simulink model "TrajectoryFollowVehicleWith14DoF"  (R2024a)
settings: Solver=VariableStepAuto  StartTime=0  StopTime=14  FixedStep=timeStep  RelTol=1e-3
PreLoadFcn:
  | useDynamicsStanley = false; %Simulink model to move according to the scenario trajectory.
  | vehicleVariant = "3DOF";
PostLoadFcn:
  | load(fullfile(matlabroot,'toolbox','driving','drivingdata','rrScenarioSimTypes.mat'));
  | helperSLTrajectoryFollowerWithRRScenarioSetup();
  | heightMap = "flat";
  | if isfile("pathFollowingUtil/gridMap_groundHeight_RT.mat")
  |     load("gridMap_groundHeight_RT.mat");
  | end
  | % if exist("z_2DTable", "var") && exist("xBreakPts", "var") && exist("yBreakPts", "var")
  | %     hegihtMap = "2DMap";
  | % end
  | % if isfile("CRG/crgRoad.crg")
  | %     crgData = crg_read('CRG/crgRoad.crg');
  | % end
InitFcn:
  | if ~exist("useLongitudinalEV", "var")
  |     useLongitudinalEV = false;
  | end
StartFcn:
  | % set_param(bdroot, 'Profile', 'on');
StopFcn:
  | % set_param(bdroot, 'Profile', 'off');
  | % slprofreport(bdroot, 'report14DoF.html');
undefined symbols (not defined in the file or in its folder): ActorRuntime, Camera, control_timeStep, Defined, DiscIntNeverNeededParam, dz, Ego, egoInitialPose, egoInitialPoseCG, egoInitialPoseRear, InitVehicle, kmph2mps, Lane, lr, m, magnitude, max_dc, n, numReferencePose, pitch, roll, RRtimeStep, SceneData, SRE, steerGear, tau, tau2, timeStep, User, VehicleData, WheelPoses, X, xBreakPts, Y, yaw, yBreakPts, Z, z_2DTable
libraries: sm_lib x108, nesl_utility x62, sm_vehicle_utilities_lib x30, simulink_extras x12, roadrunnerscenario x6, simulink x4, drivingvehiclecontroller x4, autolibshared x2, mpcadaslib x2, autolibutils x1, METI_Lib_vehicle_model x1
(part 1 of 6)
settings Model: Creator=The MathWorks, Inc.  LastModifiedBy=nobuakif
settings DataIOCC: SaveOutput=off  DSMLogging=off  InspectSignalLogs=on  SaveTime=off  ReturnWorkspaceOutputs=off
settings OptimizationCC: DefaultParameterBehavior=Inlined  ReuseModelBlockBuffer=off
settings DebuggingCC: ParameterTunabilityLossMsg=error  UnconnectedInputMsg=warning  UnconnectedOutputMsg=warning  UnconnectedLineMsg=warning
settings ModelReferenceCC: EnableRefExpFcnMdlSchedulingChecks=on  PropagateSignalLabelsOutOfModel=off
settings RTWCC: GenCodeOnly=on  GenerateReport=on  GPUComputeCapability=3.5
settings CodeAppCC: ForceParamTrailComments=on
settings GRTTargetCC: TargetLangStandard=C89/C90 (ANSI)

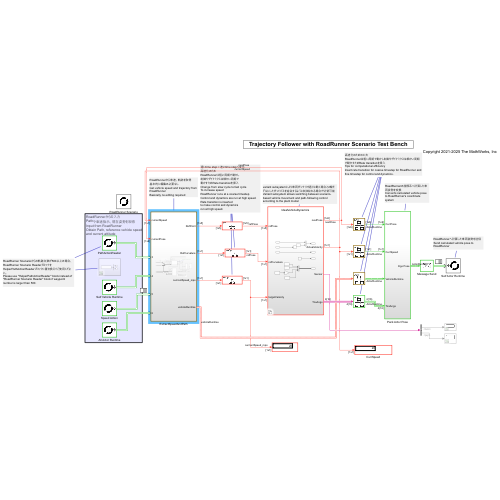
[thumbnail: Simulink's stored preview of the top-level diagram]
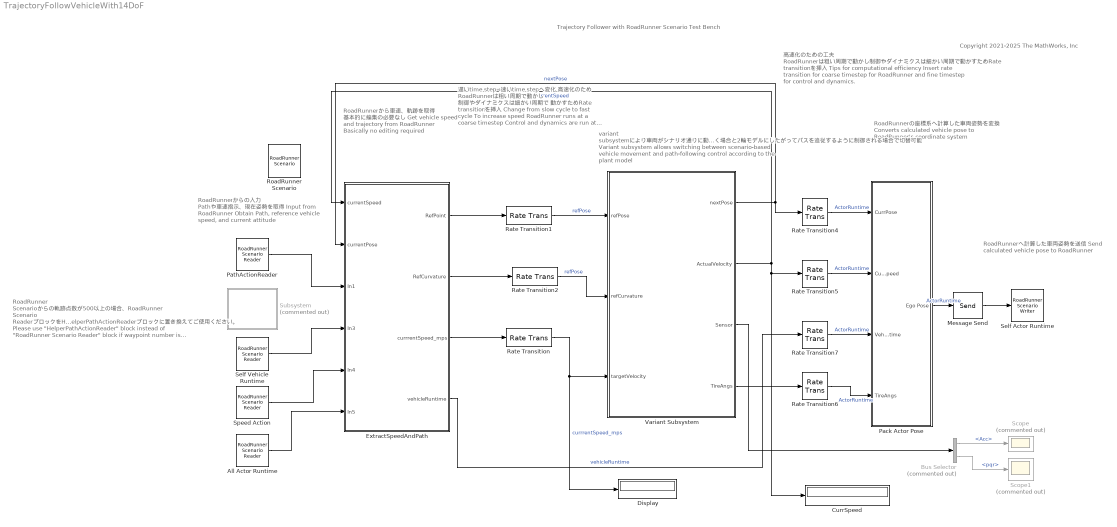
== system TrajectoryFollowVehicleWith14DoF ==
  note: 高速化のための工夫
      | RoadRunnerは粗い周期で動かし制御やダイナミクスは細かい周期で動かすためRate transitionを挿入
      | Tips for computational efficiency
      | Insert rate transition for coarse timestep for RoadRunner and fine timestep for control and dynamics.
  note: RoadRunnerからの入力
      | Pathや車速指示、現在姿勢を取得
      | Input from RoadRunner
      | Obtain Path, reference vehicle speed,
      | and current attitude
  note: Trajectory Follower with RoadRunner Scenario Test Bench
  note: Copyright 2021-2025 The MathWorks, Inc
  note: RoadRunnerへ計算した車両姿勢を送信
      | Send calculated vehicle pose to RoadRunner
  note: RoadRunnerの座標系へ計算した車両姿勢を変換
      | Converts calculated vehicle pose to RoadRunner's coordinate system
  note: variant subsystemにより車両がシナリオ通りに動く場合と2輪モデルにしたがってパスを追従するように制御される場合で切替可能
      | Variant subsystem allows switching between scenario-based vehicle movement and path-following control according to the plant model
  note: RoadRunnerから車速、軌跡を取得
      | 基本的に編集の必要なし
      | Get vehicle speed and trajectory from RoadRunner
      | Basically no editing required
  note: RoadRunner Scenarioからの軌跡点数が500以上の場合、RoadRunner Scenario ReaderブロックをHelperPathActionReaderブロックに置き換えてご使用ください。
      | Please use "HelperPathActionReader" block instead of "RoadRunner Scenario Reader" block if waypoint number is larger than 500.
  note: 遅いtime step⇒速いtime stepへ変化
      | 高速化のため
      | RoadRunnerは粗い周期で動かし
      | 制御やダイナミクスは細かい周期で
      | 動かすためRate transitionを挿入
      | Change from slow cycle to fast cycle
      | To increase speed
      | RoadRunner runs at a coarse timestep
      | Control and dynamics are run at high speed.
      | Rate transition is inserted
      | to make control and dynamics
      | run at high speed.
  All Actor Runtime : roadrunnerscenario/RoadRunner Scenario Reader  TopicCategory=Actor  ActorCategory=All Types  ActionType=Path Following  EventType=User-Defined  TopicType=Actor Pose  VehicleType=Vehicle Specifications  UserDefinedAction=Action1  UserDefinedEvent=Event1  Filter=None  SensorTopic=Target Poses  LaneBoundaryOutputTopic=Ego-Lane  SensorID=1  SampleTime=RRtimeStep
  Bus Selector : BusSelector  Commented=on  OutputSignals=IMU.Acc,IMU.pqr
  CurrSpeed : Display
  Display : Display
  ExtractSpeedAndPath : Subsystem
  Message Send : Send  OutputPortMessageModes=m
  Pack Actor Pose : Subsystem
  PathActionReader : roadrunnerscenario/RoadRunner Scenario Reader  TopicCategory=Action  ActorCategory=Vehicle  ActionType=Path Following  EventType=User-Defined  TopicType=Actor Specifications  VehicleType=Vehicle Pose  UserDefinedAction=Action1  UserDefinedEvent=Event1  Filter=Self  SensorTopic=Target Poses  LaneBoundaryOutputTopic=Ego-Lane  SensorID=1  SampleTime=RRtimeStep
  Rate Transition : RateTransition  OutPortSampleTime=timeStep
  Rate Transition1 : RateTransition  OutPortSampleTime=timeStep
  Rate Transition2 : RateTransition  OutPortSampleTime=timeStep
  Rate Transition{4..7} (4 alike) : RateTransition  OutPortSampleTime=RRtimeStep
  RoadRunner Scenario : roadrunnerscenario/RoadRunner Scenario  UserDefinedActions={}  UserDefinedEvents={}
  Scope : Scope  Commented=on
  Scope1 : Scope  Commented=on
  Self Actor Runtime : roadrunnerscenario/RoadRunner Scenario Writer  TopicCategory=Actor  ActorCategory=Vehicle  EventType=Action Complete  UserDefinedEvent=Event1  VehicleType=Vehicle Pose  TopicType=Actor Pose
  Self Vehicle Runtime : roadrunnerscenario/RoadRunner Scenario Reader  TopicCategory=Actor  ActorCategory=Vehicle  ActionType=Path Following  EventType=User-Defined  TopicType=Actor Specifications  VehicleType=Vehicle Pose  UserDefinedAction=Action1  UserDefinedEvent=Event1  Filter=Self  SensorTopic=Target Poses  LaneBoundaryOutputTopic=Ego-Lane  SensorID=1  SampleTime=RRtimeStep
  Speed Action : roadrunnerscenario/RoadRunner Scenario Reader  TopicCategory=Action  ActorCategory=All Types  ActionType=Speed Change  EventType=User-Defined  TopicType=Actor Specifications  VehicleType=Vehicle Specifications  UserDefinedAction=Action1  UserDefinedEvent=Event1  Filter=Self  SensorTopic=Target Poses  LaneBoundaryOutputTopic=Ego-Lane  SensorID=1  SampleTime=RRtimeStep
  Subsystem : Subsystem  Commented=on
  Variant Subsystem : Subsystem  Variant=on
  wires:
  Rate Transition/1 -> Display/1, Variant Subsystem/3(targetVelocity)  "currrentSpeed_mps"
  Message Send/1 -> Self Actor Runtime/1
  Rate Transition1/1 -> Variant Subsystem/1(refPose)  "refPose"
  Variant Subsystem/2(ActualVelocity) -> CurrSpeed/1, Rate Transition5/1, ExtractSpeedAndPath/1(currentSpeed)  "currentSpeed"
  Variant Subsystem/1(nextPose) -> Rate Transition4/1, ExtractSpeedAndPath/2(currentPose)  "nextPose"
  Rate Transition2/1 -> Variant Subsystem/2(refCurvature)  "refPose"
  PathActionReader/1 -> ExtractSpeedAndPath/3(In1)
  Self Vehicle Runtime/1 -> ExtractSpeedAndPath/4(In3)
  Speed Action/1 -> ExtractSpeedAndPath/5(In4)
  All Actor Runtime/1 -> ExtractSpeedAndPath/6(In5)
  ExtractSpeedAndPath/1(RefPoint) -> Rate Transition1/1
  ExtractSpeedAndPath/2(RefCurvature) -> Rate Transition2/1
  ExtractSpeedAndPath/3(currrentSpeed_mps) -> Rate Transition/1
  ExtractSpeedAndPath/4(vehicleRuntime) -> Rate Transition7/1  "vehicleRuntime"
  Variant Subsystem/3(Sensor) -> Bus Selector/1
  Bus Selector/1 -> Scope/1  "<Acc>"
  Bus Selector/2 -> Scope1/1  "<pqr>"
  Pack Actor Pose/1(Ego Pose) -> Message Send/1  "ActorRuntime"
  Variant Subsystem/4(TireAngs) -> Rate Transition6/1
  Rate Transition4/1 -> Pack Actor Pose/1(CurrPose)  "ActorRuntime"
  Rate Transition5/1 -> Pack Actor Pose/2(CurrSpeed)  "ActorRuntime"
  Rate Transition6/1 -> Pack Actor Pose/4(TireAngs)  "ActorRuntime"
  Rate Transition7/1 -> Pack Actor Pose/3(VehicleRuntime)  "ActorRuntime"

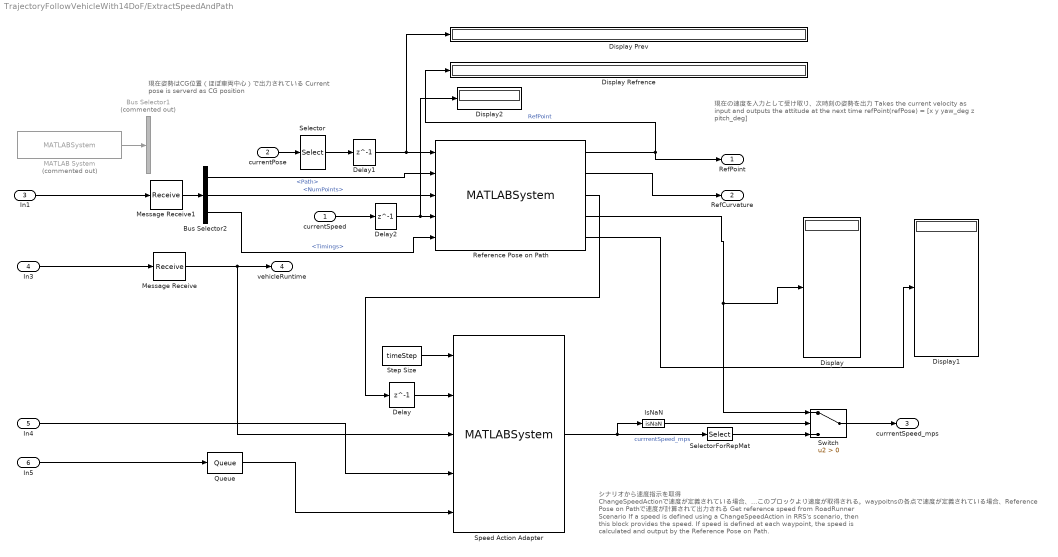
== system TrajectoryFollowVehicleWith14DoF/ExtractSpeedAndPath ==
  note: 現在の速度を入力として受け取り、次時刻の姿勢を出力
      | Takes the current velocity as input and outputs the attitude at the next time
      | refPoint(refPose) = [x y yaw_deg z pitch_deg]
  note: シナリオから速度指示を取得
      | ChangeSpeedActionで速度が定義されている場合、このブロックより速度が取得される。waypoitnsの各点で速度が定義されている場合、Reference Pose on Pathで速度が計算されて出力される
      | Get reference speed from RoadRunner Scenario
      | If a speed is defined using a ChangeSpeedAction in RRS's scenario, then this block provides the speed. If speed is defined at each waypoint, the speed is calculated and output by the Reference Pose on Path.
  note: 現在姿勢はCG位置（ほぼ車両中心）で出力されている
      | Current pose is serverd as CG position
  currentSpeed : Inport
  currentPose : Inport  Port=2
  In1 : Inport  Port=3
  In3 : Inport  Port=4
  In4 : Inport  Port=5
  In5 : Inport  Port=6
  Bus Selector1 : BusSelector  Commented=on  OutputSignals=Path,NumPoints
  Bus Selector2 : BusSelector  OutputSignals=PathTarget.Path,PathTarget.NumPoints,PathTarget.Timings
  Delay : Delay  DelayLength=1  InitialCondition=logical(0)
  Delay1 : Delay  DelayLength=1  InitialCondition=egoInitialPoseCG.CurrPose
  Delay2 : Delay  DelayLength=1  InitialCondition=norm(egoInitialPose.Velocity)
  Display : Display
  Display Prev : Display
  Display Refrence : Display
  Display1 : Display
  Display2 : Display
  IsNaN : RelationalOperator  Operator=isNaN  OutDataTypeStr=boolean  RndMeth=Simplest  InputSameDT=off
  MATLAB System : MATLABSystem  Commented=on  System=HelperPathActionReader  sampleTime=-1
      mask Type: HelperPathActionReader
      mask Display:
      | disp('HelperPathActionReader');
      | port_label('output',1,'PathTarget');
  Message Receive : Receive  InputPortMessageModes=m
  Message Receive1 : Receive  InputPortMessageModes=m
  Queue : Queue  InputPortMessageModes=m  OutputPortMessageModes=m  OverwriteOldest=on  Capacity=16  QueueType=LIFO
  Reference Pose on Path : MATLABSystem  System=HelperReferencePoseOnPath  timeStep=timeStep  refPointSpeedOffset=useDynamicsStanley == false  refPts_offset=refPts_offset  output_offset=0  debugFig=true  saveFigVideo=false  zoomFig=10  searchIndx=10  numReferencePose=numReferencePose  controlTimestep=0.1
      mask Type: HelperReferencePoseOnPath
      mask Display:
      | disp(['HelperReferencePoseOnPath' char(10) '' char(10) '' char(10) '' char(10) '']);
      | port_label('input',1,'PrevVehicleInfo');
      | port_label('input',2,'Trajectory');
      | port_label('input',3,'NumTrajPoints');
      | port_label('input',4,'currentSpeed');
      | port_label('input',5,'Traj_timings');
      | port_label('output',1,'RefPointOnPath');
      | port_label('output',2,'RefCurvature');
      | port_label('output',3,'IsGoalReached');
      | port_label('output',4,'RefSpeedOnPath');
      | port_label('output',5,'RefTimings');
  Selector : Selector  InputPortWidth=6  IndexOptions=Index vector (dialog)  Indices=1:5  OutputSizes=1
  SelectorForRepMat : Selector  InputPortWidth=1  IndexOptions=Index vector (dialog)  Indices=ones(numReferencePose, 1)  OutputSizes=1
  Speed Action Adapter : MATLABSystem  InputPortMessageModes=n,n,n,m,m  System=HelperSpeedActionAdapter
      mask Type: HelperSpeedActionAdapter
      mask Display:
      | disp(['HelperSpeedActionAdapter' char(10) '' char(10) '']);
      | port_label('input',1,'timestep');
      | port_label('input',2,'stopVehicle');
      | port_label('input',3,'vehicleRuntime');
      | port_label('input',4,'msgSpeedAction');
      | port_label('input',5,'msgAllVehicleRuntime');
      | port_label('output',1,'currentSpeed');
  Step Size : Constant  Value=timeStep
  Switch : Switch  Criteria=u2 > Threshold  SaturateOnIntegerOverflow=off  InputSameDT=off
  RefPoint : Outport
  RefCurvature : Outport  Port=2
  currrentSpeed_mps : Outport  Port=3
  vehicleRuntime : Outport  Port=4
  wires:
  Delay/1 -> Speed Action Adapter/2
  Reference Pose on Path/1 -> RefPoint/1, Display Refrence/1  "RefPoint"
  Step Size/1 -> Speed Action Adapter/1
  Message Receive1/1 -> Bus Selector2/1
  Reference Pose on Path/3 -> Delay/1
  Bus Selector2/1 -> Reference Pose on Path/2  "<Path>"
  Message Receive/1 -> vehicleRuntime/1, Speed Action Adapter/3
  In4/1 -> Speed Action Adapter/4
  Bus Selector2/2 -> Reference Pose on Path/3  "<NumPoints>"
  In3/1 -> Message Receive/1
  Reference Pose on Path/2 -> RefCurvature/1
  In5/1 -> Queue/1
  Speed Action Adapter/1 -> SelectorForRepMat/1, IsNaN/1  "currrentSpeed_mps"
  In1/1 -> Message Receive1/1
  currentSpeed/1 -> Delay2/1
  Queue/1 -> Speed Action Adapter/5
  Delay1/1 -> Reference Pose on Path/1, Display Prev/1
  currentPose/1 -> Selector/1
  Selector/1 -> Delay1/1
  Delay2/1 -> Reference Pose on Path/4, Display2/1
  MATLAB System/1 -> Bus Selector1/1
  Bus Selector2/3 -> Reference Pose on Path/5  "<Timings>"
  Reference Pose on Path/4 -> Switch/1, Display/1
  Reference Pose on Path/5 -> Display1/1
  Switch/1 -> currrentSpeed_mps/1
  IsNaN/1 -> Switch/2
  SelectorForRepMat/1 -> Switch/3

== system TrajectoryFollowVehicleWith14DoF/Pack Actor Pose ==
  CurrPose : Inport
  CurrSpeed : Inport  Port=2
  VehicleRuntime : Inport  Port=3  OutDataTypeStr=Bus: BusVehicleRuntime
  TireAngs : Inport  Port=4
  Assign : BusAssignment  AssignedSignals=ActorRuntime.Pose,ActorRuntime.Velocity,WheelPoses
  Bus Selector : BusSelector  Commented=on  OutputSignals=ActorRuntime
  Bus Selector1 : BusSelector  OutputSignals=WheelPoses
  Bus Selector2 : BusSelector  OutputSignals=roll,pitch,yaw,dz
  Cvt2RRSCoodinate : MATLAB Function  TreatAsAtomicUnit=on
  Display : Display
  Gain1 : Gain
  MATLAB Function : MATLAB Function  Commented=on  TreatAsAtomicUnit=on
  MATLAB System : MATLABSystem  System=packWheelPoses  SimulateUsing=Code generation
      mask Type: packWheelPoses
      mask Display:
      | disp('packWheelPoses');
      | port_label('input',1,'wheelPosesPrev');
      | port_label('input',2,'roll');
      | port_label('input',3,'pitch');
      | port_label('input',4,'yaw');
      | port_label('input',5,'dz');
      | port_label('output',1,'wheelPoses');
  Pose Generation : MATLAB Function  TreatAsAtomicUnit=on
  Selector : Selector  InputPortWidth=6  IndexOptions=Index vector (dialog)  Indices=[3, 5]  OutputSizes=1
  Terminator : Terminator  Commented=on
  Velocity XYZ Components : MATLAB Function  TreatAsAtomicUnit=on
  Ego Pose : Outport
  wires:
  Bus Selector/1 -> Terminator/1  "<ActorRuntime>"
  Bus Selector2/3 -> MATLAB System/4  "<yaw>"
  TireAngs/1 -> Bus Selector2/1
  Bus Selector2/2 -> MATLAB System/3  "<pitch>"
  Bus Selector2/1 -> MATLAB System/2  "<roll>"
  VehicleRuntime/1 -> Assign/1, Bus Selector1/1
  CurrPose/1 -> Selector/1, Cvt2RRSCoodinate/1(pose)
  Bus Selector2/4 -> Gain1/1  "<dz>"
  Cvt2RRSCoodinate/1(RRSPose) -> Pose Generation/1(pose)
  Selector/1 -> Velocity XYZ Components/1(yaw_pitch)
  Assign/1 -> Ego Pose/1
  Bus Selector1/1 -> MATLAB System/1  "<WheelPoses>"
  CurrSpeed/1 -> Velocity XYZ Components/2(speed)
  Gain1/1 -> MATLAB System/5
  Pose Generation/1(currPose) -> Assign/2  "Pose"
  Velocity XYZ Components/1(velocity) -> Assign/3, Display/1  "Velocity"
  MATLAB System/1 -> Assign/4

== system TrajectoryFollowVehicleWith14DoF/Subsystem ==
  Bus Selector2 : BusSelector  OutputSignals=PathTarget.Path,PathTarget.NumPoints
  MATLAB System : MATLABSystem  System=HelperPathActionReader  sampleTime=-1
      mask Type: HelperPathActionReader
      mask Display:
      | disp('HelperPathActionReader');
      | port_label('output',1,'PathTarget');
  Terminator1 : Terminator
  Terminator2 : Terminator
  wires:
  Bus Selector2/2 -> Terminator2/1  "<NumPoints>"
  MATLAB System/1 -> Bus Selector2/1
  Bus Selector2/1 -> Terminator1/1  "<Path>"

== system TrajectoryFollowVehicleWith14DoF/Variant Subsystem ==
  refPose : Inport
  refCurvature : Inport  Port=2
  targetVelocity : Inport  Port=3
  IdealVehicleDynamics : Subsystem  VariantControl="useDynamicsStanley == false  && useLongitudinalEV == false"
  LongitudinalEV : Subsystem  VariantControl=useDynamicsStanley == false && useLongitudinalEV == true
  StanleyControl_vehicleDynamics : Subsystem  VariantControl="useDynamicsStanley == true  && useLongitudinalEV == false"
  nextPose : Outport
  ActualVelocity : Outport  Port=2
  Sensor : Outport  Port=3
  TireAngs : Outport  Port=4

== system TrajectoryFollowVehicleWith14DoF/Variant Subsystem/IdealVehicleDynamics ==
  refPose : Inport
  refCurvature : Inport  Port=2
  targetVelocity : Inport  Port=3
  Bus Creator : BusCreator  Inputs=4
  Constant : Constant  Value=zeros(4,1)
  Constant2 : Constant  Value=zeros(4,1)
  Constant3 : Constant  Value=zeros(4,1)
  Gain : Gain
  Ground : Ground
  Terminator : Terminator
  Vector Concatenate : Concatenate
  Zero : Constant  Value=0  OutDataTypeStr=Inherit: Inherit via back propagation
  dz : Constant  Value=zeros(4,1)
  nextPose : Outport
  ActualVelocity : Outport  Port=2
  Sensor : Outport  Port=3
  TireAngs : Outport  Port=4
  wires:
  targetVelocity/1 -> ActualVelocity/1
  refCurvature/1 -> Terminator/1
  refPose/1 -> Vector Concatenate/1
  Vector Concatenate/1 -> nextPose/1
  Zero/1 -> Vector Concatenate/2
  Constant3/1 -> Gain/1  "constnt"
  Constant/1 -> Bus Creator/1  "roll"
  Constant2/1 -> Bus Creator/2  "pitch"
  Gain/1 -> Bus Creator/3  "yaw"
  Bus Creator/1 -> TireAngs/1
  Ground/1 -> Sensor/1
  dz/1 -> Bus Creator/4  "dz"

== system TrajectoryFollowVehicleWith14DoF/Variant Subsystem/LongitudinalEV ==
  note: Same as Ideal movement
  refPose : Inport
  refCurvature : Inport  Port=2
  targetVelocity : Inport  Port=3
  Bus Creator : BusCreator  Inputs=4
  Constant : Constant  Value=zeros(4,1)
  Constant2 : Constant  Value=zeros(4,1)
  Constant3 : Constant  Value=zeros(4,1)
  Gain : Gain
  Ground : Ground
  Selector : Selector  InputPortWidth=5  IndexOptions=Index vector (dialog)  Indices=4  OutputSizes=1
  Terminator : Terminator
  VDBS_PTBS : Subsystem  VariantControl=true
  Vector Concatenate : Concatenate
  Zero : Constant  Value=0  OutDataTypeStr=Inherit: Inherit via back propagation
  dz : Constant  Value=zeros(4,1)
  nextPose : Outport
  ActualVelocity : Outport  Port=2
  Sensor : Outport  Port=3
  TireAngs : Outport  Port=4
  wires:
  Ground/1 -> Sensor/1
  refCurvature/1 -> Terminator/1
  dz/1 -> Bus Creator/4  "dz"
  Constant2/1 -> Bus Creator/2  "pitch"
  refPose/1 -> Selector/1, Vector Concatenate/1
  Vector Concatenate/1 -> nextPose/1
  Constant3/1 -> Gain/1  "constnt"
  Bus Creator/1 -> TireAngs/1
  Zero/1 -> Vector Concatenate/2
  Constant/1 -> Bus Creator/1  "roll"
  targetVelocity/1 -> VDBS_PTBS/1(tgt_speed_mps)
  Gain/1 -> Bus Creator/3  "yaw"
  VDBS_PTBS/1(act_speed_mps) -> ActualVelocity/1  "speed_mps"
  Selector/1 -> VDBS_PTBS/2(slope_degree)

== system TrajectoryFollowVehicleWith14DoF/Variant Subsystem/StanleyControl_vehicleDynamics ==
  note: 車両ダイナミクスブロック
      | 2輪モデル、14自由度のフルビークルモデル、Simscape Multibodyでのフルビークルモデルを切り替えて使用可能
      | Vehicle Dynamics Block
      | Switch between bicycle models, full vehicle models with 14 degrees of freedom, and full vehicle models with Simscape Multibody
  note: 制御ブロック
      | 参照軌跡と参照車速に収束するようにステアリング角度、加速指示、減速指示を出力
      | Control block
      | Outputs steering angle, acceleration instructions, and deceleration instructions to converge with reference trajectory and reference vehicle speed
  note: bicycleモデルの場合、z値やピッチの情報がないためRoadRunner Sceanrioからの参照値を追加
      | For bicycle models, add reference values from RoadRunner Sceanrio as there is no z-value or pitch information
  refPose : Inport
  refCurvature : Inport  Port=2
  targetVelocity : Inport  Port=3
  Bus Selector : BusSelector  OutputSignals=CurrPose
  Bus Selector2 : BusSelector  Commented=on  OutputSignals=CurrPose
  Delay1 : Delay  DelayLength=1  InitialCondition=egoInitialPoseRear
  Lateral Metrics : MATLAB Function  Commented=on  TreatAsAtomicUnit=on
  Override Z and Pitch : Subsystem  Variant=on
  Stanley Controller : Subsystem  Commented=on
  Terminator : Terminator  Commented=on
  Terminator1 : Terminator  Commented=on
  Variant Subsystem : Subsystem  Variant=on
  Vehicle Dynamics1 : Subsystem  Variant=on  VariantControl=Vehicle Dynamics
  nextPose : Outport
  ActualVelocity : Outport  Port=2
  Sensor : Outport  Port=3
  TireAngs : Outport  Port=4
  wires:
  Vehicle Dynamics1/1(VehicleInfoRear) -> Delay1/1
  Vehicle Dynamics1/2(Speed) -> ActualVelocity/1  "speed"
  Bus Selector/1 -> Override Z and Pitch/1(currPose)  "<CurrPose>"
  Lateral Metrics/2(headingError) -> Terminator1/1  "relative_heading"
  Bus Selector2/1 -> Lateral Metrics/1(currPose)  "<CurrPose>"
  Lateral Metrics/1(positionError) -> Terminator/1  "position_error"
  Vehicle Dynamics1/4(TireAngs) -> TireAngs/1
  Override Z and Pitch/1(Out1) -> Bus Selector2/1, nextPose/1
  [refPose] -> Override Z and Pitch/2(refPose)
  Vehicle Dynamics1/3(VehicleInfoCG) -> Bus Selector/1
  Delay1/1 -> Variant Subsystem/1(VehicleInfo)
  refPose/1 -> Variant Subsystem/2(RefPose), [refPose]
  refCurvature/1 -> Variant Subsystem/3(Curvature)
  targetVelocity/1 -> Variant Subsystem/4(Speed)
  Variant Subsystem/1(SteerCmd) -> Vehicle Dynamics1/1(Steering Angle)
  Variant Subsystem/2(AccelCmd) -> Vehicle Dynamics1/2(Acceleration)
  Variant Subsystem/3(DecelCmd) -> Vehicle Dynamics1/3(Deceleration)
  Vehicle Dynamics1/5(Sensors) -> Sensor/1

== system TrajectoryFollowVehicleWith14DoF/Variant Subsystem/LongitudinalEV/VDBS_PTBS ==
  tgt_speed_mps : Inport
  slope_degree : Inport  Port=2
  Bus Selector : BusSelector  Commented=on  OutputSignals=Veh.xdot
  Controllers : Subsystem  Commented=on
      mask Display: image('SystemControllers.png','center')
  Environment : Subsystem  Commented=on
      mask Display: disp(getString(message('autoblks:autoblkVehMask:environ')))
  Longitudinal Driver : Subsystem  Commented=on  Variant=on  VariantControlMode=label  VariantControl=Variant1  LabelModeActiveChoice=0
      mask Display:
      | if strcmp('1',get_param(gcb,'ActiveVariant'))
      |     disp('Open Loop')
      | else
      |     image('LongitudinalDriver.png','center');
      | end
  Model : ModelReference  ModelNameDialog=EV_PowerTrain.slx  SimulationMode=Normal  ModelReferenceVersion=1.7
      settings: PortSchema="{\"entries\":[{\"content\":{\"sides\":[{\"content\":{\"connectorIds\":[\"In2\",\"In1\"]},\"type\":\"ConnectorPlacement.EquallySpacedRectSide\",\"uuid\":\"f2ffd824-f876-47cf-a2eb-b1f532355f92\"},{\"content\":{\"connectorIds\":[\"Out1\"],\"side\":\"RIGHT\"},\"type\":\"ConnectorPlacement.EquallySpacedRectSide\",\"uuid\":\"21b29aa8-3d5b-4060-b5a1-b1d2085b4ec6\"},{\"content\":{\"side\":\"TOP\"},\"type\":\"ConnectorPlacement.EquallySpacedRectSide\",\"uuid\":\"fa1fab69-2b9c-4691-81d7-0efb385da189\"}]},\"type\":\"ConnectorPlacement.EquallySpacedConnector\",\"uuid\":\"fa8fdda2-0c38-4013-b276-2892146cce54\"}],\"packageUris\":[\"http://schema.mathworks.com/mf0/Connector/R2020b\"],\"version\":\"1.0\"}"
  Passenger Car : Subsystem  Commented=on
      mask Display: image('PassengerVehicle.png','center')
  Rate Transition : RateTransition  OutPortSampleTime=timeStep
  Rate Transition1 : RateTransition  OutPortSampleTime=timeStep
  Saturation : Saturate  Commented=on  UpperLimit=inf  LowerLimit=0
  Unit Delay : UnitDelay  Commented=on  SampleTime=-1  HasFrameUpgradeWarning=on
  Visualization : Subsystem  Commented=on
      mask Display: disp(getString(message('autoblks:autoblkVehMask:visual')))
  act_speed_mps : Outport
  wires:
  Controllers/1(Ctrl) -> Passenger Car/2(Ctrl)
  tgt_speed_mps/1 -> Rate Transition1/1, Longitudinal Driver/1("Vref "), Visualization/2(VelocityRef)
  Longitudinal Driver/1(" OpCmds") -> Controllers/2(OpCmds)
  Passenger Car/1(VehPlnt) -> Bus Selector/1, Longitudinal Driver/2("Vfdbk "), Controllers/3(VehPlnt), Visualization/1(Veh Bus)
  Environment/1(Environment) -> Controllers/1(Env), Passenger Car/1(Env)
  slope_degree/1 -> Rate Transition/1, Environment/1(slope_deg)
  Bus Selector/1 -> Unit Delay/1  "<xdot>"
  Unit Delay/1 -> Saturation/1
  Saturation/1 -> ?
  Model/1 -> act_speed_mps/1
  Rate Transition/1 -> Model/2
  Rate Transition1/1 -> Model/1

== system TrajectoryFollowVehicleWith14DoF/Variant Subsystem/StanleyControl_vehicleDynamics/Override Z and Pitch ==
  note: 1) Add Subsystem or Model blocks as valid variant choices.
      | 2) You cannot connect blocks at this level. At simulation, connectivity is automatically
      | determined, based on the active variant and port name matching.
  currPose : Inport
  refPose : Inport  Port=2
  notOverride : Subsystem  VariantControl="vehicleVariant == \"14DOF\" || vehicleVariant == \"Multibody\""
  override : Subsystem  VariantControl="vehicleVariant == \"3DOF\""
  Out1 : Outport

== system TrajectoryFollowVehicleWith14DoF/Variant Subsystem/StanleyControl_vehicleDynamics/Stanley Controller ==
  note: x, y, yaw, z, pitch
  In Bus Element : Inport  PortName=VehicleInfo  Element=CurrPose
  In Bus Element1 : Inport  PortName=VehicleInfo  Element=CurrVelocity
  In Bus Element2 : Inport  PortName=VehicleInfo  Element=CurrYawRate
  In Bus Element3 : Inport  PortName=VehicleInfo  Element=CurrSteer
  RefPose : Inport  Port=2
  Curvature : Inport  Port=3
  Speed : Inport  Port=4
  Constant1 : Constant
  Constant2 : Constant
  Constant3 : Constant  Value=0
  Display{,3..5} (4 alike) : Display
  DisplayCurrPose : Display
  DisplayCurrPose1 : Display
  DisplayRefPose : Display
  Lateral Controller Stanley : drivingvehiclecontroller/Lateral Controller Stanley  ModelType=Dynamic bicycle model  PositionGainF=3  PositionGainR=2.5  YawRateGain=0.2  DelayGain=0.2  VehicleMass=m  Lf=lf  Lr=lr  TireStiffness=Cf  Wheelbase=2.8  MaxSteeringAngle=steerLimit
  Longitudinal Controller Stanley : drivingvehiclecontroller/Longitudinal Controller Stanley  Kp=2  Ki=1  SampleTime=timeStep  MaxAcceleration=max_ac  MaxDeceleration=max_dc
  Selector : Selector  InputPortWidth=5  IndexOptions=Index vector (dialog)  Indices=[1:3]  OutputSizes=1
  Selector1 : Selector  InputPortWidth=5  IndexOptions=Index vector (dialog)  Indices=[1:3]  OutputSizes=1
  SteerCmd : Outport
  AccelCmd : Outport  Port=2
  DecelCmd : Outport  Port=3
  wires:
  In Bus Element/1 -> DisplayCurrPose/1, Selector1/1
  Lateral Controller Stanley/1 -> Display/1, SteerCmd/1
  In Bus Element2/1 -> Display4/1
  In Bus Element1/1 -> DisplayCurrPose1/1, Lateral Controller Stanley/3, Longitudinal Controller Stanley/2
  Constant1/1 -> Longitudinal Controller Stanley/3
  Longitudinal Controller Stanley/2 -> DecelCmd/1
  Constant2/1 -> Lateral Controller Stanley/4
  In Bus Element3/1 -> Display5/1
  Constant3/1 -> Longitudinal Controller Stanley/4
  RefPose/1 -> DisplayRefPose/1, Selector/1
  Longitudinal Controller Stanley/1 -> AccelCmd/1
  Curvature/1 -> Display3/1
  Speed/1 -> Longitudinal Controller Stanley/1
  Selector/1 -> Lateral Controller Stanley/1
  Selector1/1 -> Lateral Controller Stanley/2

== system TrajectoryFollowVehicleWith14DoF/Variant Subsystem/StanleyControl_vehicleDynamics/Variant Subsystem ==
  note: 1) Add Subsystem or Model blocks as valid variant choices.
      | 2) You cannot connect blocks at this level. At simulation, connectivity is automatically
      | determined, based on the active variant and port name matching.
  VehicleInfo : Inport
  RefPose : Inport  Port=2
  Curvature : Inport  Port=3
  Speed : Inport  Port=4
  MPC : Subsystem  VariantControl="controlMode == \"mpc\""
  Stanley : Subsystem  VariantControl="controlMode == \"stanley\""
  mpc_mod : ModelReference  ModelNameDialog=mpc_pathFollowingMod.slx  SimulationMode=Normal  VariantControl="controlMode == \"mpc_mod\""  ModelReferenceVersion=1.91
  SteerCmd : Outport
  AccelCmd : Outport  Port=2
  DecelCmd : Outport  Port=3

== system TrajectoryFollowVehicleWith14DoF/Variant Subsystem/StanleyControl_vehicleDynamics/Vehicle Dynamics1 ==
  Steering Angle : Inport
  Acceleration : Inport  Port=2
  Deceleration : Inport  Port=3
  Vehicle Dynamics 14DOF : Subsystem  VariantControl="vehicleVariant == \"14DOF\""
  Vehicle Dynamics 3DOF : Subsystem  VariantControl="vehicleVariant == \"3DOF\""
  Vehicle Dynamics Multibody : Subsystem  VariantControl="vehicleVariant == \"Multibody\""
  VehicleInfoRear : Outport
  Speed : Outport  Port=2
  VehicleInfoCG : Outport  Port=3
  TireAngs : Outport  Port=4
  Sensors : Outport  Port=5

== system TrajectoryFollowVehicleWith14DoF/Variant Subsystem/LongitudinalEV/VDBS_PTBS/Controllers ==
  Env : Inport
  OpCmds : Inport  Port=2
  VehPlnt : Inport  Port=3
  Powertrain Control Input : Subsystem
  Powertrain Control Module (PCM) : Subsystem
  Powertrain Control Output : Subsystem
  Terminator : Terminator
  Ctrl : Outport  VectorParamsAs1DForOutWhenUnconnected=off
  wires:
  [PtCtrl] -> Ctrl/1
  Env/1 -> Terminator/1
  [OpCmds] -> Powertrain Control Input/1(OpCmds)
  Powertrain Control Output/1(PtCtrl) -> [PtCtrl]
  [VehPlnt] -> Powertrain Control Input/2(VehPlnt)
  VehPlnt/1 -> [VehPlnt]
  OpCmds/1 -> [OpCmds]
  Powertrain Control Input/1(AccelPdl) -> Powertrain Control Module (PCM)/1(AccCmd)
  Powertrain Control Input/2(DecelPdl) -> Powertrain Control Module (PCM)/2(DecCmd)
  Powertrain Control Input/3(VehSpdFdbk) -> Powertrain Control Module (PCM)/3(VehSpdFdbk)
  Powertrain Control Input/4(MotSpd) -> Powertrain Control Module (PCM)/4(MotSpd)
  Powertrain Control Module (PCM)/1(MotTrqCmd) -> Powertrain Control Output/1(MotTrqCmd)
  Powertrain Control Module (PCM)/2(BrakeCmd) -> Powertrain Control Output/2(BrkCmd)
  Powertrain Control Input/5(BMS_Sensors) -> Powertrain Control Module (PCM)/5(BMS_Sensors)
  Powertrain Control Module (PCM)/3(BMS_Info) -> Powertrain Control Output/3(BMS_Info)
  Powertrain Control Module (PCM)/4(BMS_Cmd) -> Powertrain Control Output/4(BMS_Cmd)

== system TrajectoryFollowVehicleWith14DoF/Variant Subsystem/LongitudinalEV/VDBS_PTBS/Environment ==
  slope_deg : Inport
  Bus Creator : BusCreator  Inputs=4
  Bus Creator3 : BusCreator  Inputs=3
  Bus Creator4 : BusCreator  Inputs=2
  Bus Creator5 : BusCreator  Inputs=2
  Constant3 : Constant  Value=0
  Constant6 : Constant  Value=300
  Constant7 : Constant  Value=101325
  Ground{,1..3} (4 alike) : Ground
  Environment : Outport  VectorParamsAs1DForOutWhenUnconnected=off
  wires:
  Ground2/1 -> Bus Creator5/1  "lam_mu_x"
  Ground3/1 -> Bus Creator5/2  "lam_mu_y"
  Bus Creator5/1 -> Bus Creator4/2  "Ground_mu"
  Bus Creator4/1 -> Bus Creator/3  "Ground"
  Bus Creator3/1 -> Bus Creator/4  "Wind"
  Constant3/1 -> Bus Creator3/1  "wind_x"
  Ground/1 -> Bus Creator3/2  "wind_y"
  Ground1/1 -> Bus Creator3/3  "wind_z"
  Constant6/1 -> Bus Creator/1  "Temp"
  slope_deg/1 -> Bus Creator4/1  "Grade"
  Bus Creator/1 -> Environment/1  "Environment"
  Constant7/1 -> Bus Creator/2  "Baro"

== system TrajectoryFollowVehicleWith14DoF/Variant Subsystem/LongitudinalEV/VDBS_PTBS/Longitudinal Driver ==
  note: To switch variants, right-click on this subsystem (from one level above) and chose:
      | Variant, Active choice, <your selection>
  "Vref " : Inport
  "Vfdbk " : Inport  Port=2
  Longitudinal Driver : Subsystem  VariantControl=0
      mask Display: image('LongitudinalDriver.png', 'center')
  Open Loop : Subsystem  VariantControl=1
      mask Display: disp('Open Loop')
  " OpCmds" : Outport  VectorParamsAs1DForOutWhenUnconnected=off

== system TrajectoryFollowVehicleWith14DoF/Variant Subsystem/LongitudinalEV/VDBS_PTBS/Passenger Car ==
  Env : Inport
  Ctrl : Inport  Port=2
  Bus Creator : BusCreator  Inputs=2
  Drivetrain : ModelReference  ModelNameDialog=DrivetrainEv.slx  ModelReferenceVersion=10.4
  Drivetrain Output : Subsystem
  Drivetrain Plant Input : Subsystem
  Electric Plant : Subsystem  Variant=on  VariantControlMode=label  VariantControl=Choice  LabelModeActiveChoice=Powertrain Blockset
  Electric Plant Input : Subsystem
  Electric Plant Output : Subsystem
  VehPlnt : Outport  VectorParamsAs1DForOutWhenUnconnected=off
  wires:
  Ctrl/1 -> [Ctrl]
  Env/1 -> [Env], Electric Plant Input/3(Env)
  [Ctrl] -> Drivetrain Plant Input/1(Ctrl)
  Bus Creator/1 -> VehPlnt/1
  [VehFdbk] -> Bus Creator/2  "Veh"
  Drivetrain Output/1(VehFdbk) -> [VehFdbk]
  Electric Plant Output/1(ElecFdbk) -> [ElecFdbk]
  [ElecFdbk] -> Bus Creator/1  "Elec"
  [Ctrl] -> Electric Plant Input/1(Ctrl)
  [ElecFdbk] -> Drivetrain Plant Input/2(ElecFdbk)
  [VehFdbk] -> Electric Plant Input/2(Veh)
  Drivetrain Plant Input/2(BrkCmd) -> Drivetrain/2
  Drivetrain Plant Input/1(MotTrq) -> Drivetrain/1
  Drivetrain/2 -> Drivetrain Output/2(MotSpd)
  Drivetrain/1 -> Drivetrain Output/1(VehSpd)
  [Env] -> Drivetrain Plant Input/3(Env)
  Drivetrain Plant Input/3(Grade) -> Drivetrain/3
  Drivetrain Plant Input/4(WindVel) -> Drivetrain/4
  Electric Plant Input/1(MotTrqCmd) -> Electric Plant/1(MotTrqCmd)
  Electric Plant Input/2(MotSpd) -> Electric Plant/2(MotSpd)
  Electric Plant Input/3(AmbTmp) -> Electric Plant/3(AmbTmp)
  Electric Plant/2(BattPwr) -> Electric Plant Output/2(BattPwr)
  Electric Plant/3(BattCrnt) -> Electric Plant Output/3(BattCrnt)
  Electric Plant/4(MotTrq) -> Electric Plant Output/4(MotTrq)
  Electric Plant/5(BMS_Sensors) -> Electric Plant Output/5(BMS_Sensors)
  Electric Plant Input/4(BMS_Info) -> Electric Plant/4(BMS_Info)
  Electric Plant Input/5(BMS_Cmd) -> Electric Plant/5(BMS_Cmd)
  Electric Plant Input/6(VehSpd) -> Electric Plant/6(VehSpd)
  Electric Plant/1(BattSoc) -> Electric Plant Output/1(BattSoc)

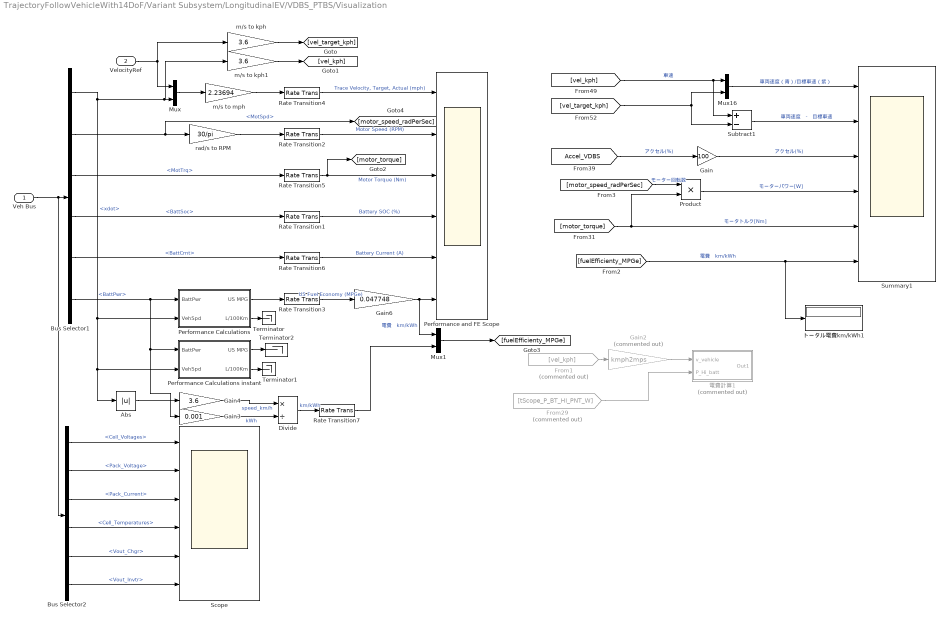
== system TrajectoryFollowVehicleWith14DoF/Variant Subsystem/LongitudinalEV/VDBS_PTBS/Visualization ==
  Veh Bus : Inport
  VelocityRef : Inport  Port=2
  Abs : Abs  SaturateOnIntegerOverflow=off
  Bus Selector1 : BusSelector  OutputSignals=Veh.xdot,Veh.MotSpd,Elec.MotTrq,Elec.BattSoc,Elec.BattCrnt,Elec.BattPwr
  Bus Selector2 : BusSelector  OutputSignals=Elec.BMS_Sensors.Cell_Voltages,Elec.BMS_Sensors.Pack_Voltage,Elec.BMS_Sensors.Pack_Current,Elec.BMS_Sensors.Cell_Temperatures,Elec.BMS_Sensors.Vout_Chgr,Elec.BMS_Sensors.Vout_Invtr
  Divide : Product  Inputs=*/
  From1 : From  Commented=on  GotoTag=vel_kph
  From29 : From  Commented=on  GotoTag=tScope_P_BT_HI_PNT_W  TagVisibility=global
  Gain : Gain  Gain=100
  Gain2 : Gain  Commented=on  Gain=kmph2mps
  Gain3 : Gain  Gain=0.001
  Gain4 : Gain  Gain=3.6
  Gain6 : Gain  Gain=0.047748
  Mux : Mux  Inputs=2
  Mux1 : Mux  Inputs=2
  Mux16 : Mux  Inputs=2
  Performance Calculations : Subsystem
  Performance Calculations instant : Subsystem
  Performance and FE Scope : Scope  NumInputPorts=6
  Product : Product
  Rate Transition{1..7} (7 alike) : RateTransition  Deterministic=off
  Scope : Scope  NumInputPorts=6
  Subtract1 : Sum  Inputs=+-
  Summary1 : Scope  NumInputPorts=6
  Terminator : Terminator
  Terminator1 : Terminator
  Terminator2 : Terminator
  m/s to kph : Gain  Gain=3.6
  m/s to kph1 : Gain  Gain=3.6
  m/s to mph : Gain  Gain=2.23694
  rad/s to RPM : Gain  Gain=30/pi
  トータル電費km/kWh1 : Display
  電費計算1 : Subsystem  Commented=on
  wires:
  Veh Bus/1 -> Bus Selector2/1, Bus Selector1/1
  Bus Selector1/1 -> Performance Calculations/2(VehSpd), Abs/1, Performance Calculations instant/2(VehSpd), m/s to kph1/1, Mux/2  "<xdot>"
  Mux/1 -> m/s to mph/1
  Performance Calculations/1(US MPG) -> Rate Transition3/1
  Performance Calculations/2(L/100Km) -> Terminator/1
  m/s to mph/1 -> Rate Transition4/1
  Bus Selector1/4 -> Rate Transition1/1  "<BattSoc>"
  VelocityRef/1 -> Mux/1, m/s to kph/1
  Rate Transition1/1 -> Performance and FE Scope/4  "Battery SOC (%)"
  Rate Transition2/1 -> Performance and FE Scope/2  "Motor Speed (RPM)"
  Rate Transition4/1 -> Performance and FE Scope/1  "Trace Velocity, Target, Actual (mph)"
  Bus Selector1/2 -> [motor_speed_radPerSec], rad/s to RPM/1  "<MotSpd>"
  Bus Selector1/6 -> Performance Calculations instant/1(BattPwr), Gain3/1, Performance Calculations/1(BattPwr)  "<BattPwr>"
  rad/s to RPM/1 -> Rate Transition2/1
  Bus Selector1/3 -> Rate Transition5/1  "<MotTrq>"
  Rate Transition5/1 -> [motor_torque], Performance and FE Scope/3  "Motor Torque (Nm)"
  Rate Transition6/1 -> Performance and FE Scope/5  "Battery Current (A)"
  Bus Selector1/5 -> Rate Transition6/1  "<BattCrnt>"
  Rate Transition3/1 -> Gain6/1  "US Fuel Economy (MPGe)"
  Bus Selector2/1 -> Scope/1  "<Cell_Voltages>"
  Bus Selector2/2 -> Scope/2  "<Pack_Voltage>"
  Bus Selector2/3 -> Scope/3  "<Pack_Current>"
  Bus Selector2/4 -> Scope/4  "<Cell_Temperatures>"
  Bus Selector2/5 -> Scope/5  "<Vout_Chgr>"
  Bus Selector2/6 -> Scope/6  "<Vout_Invtr>"
  [vel_kph] -> Subtract1/1, Mux16/1  "車速"
  [motor_torque] -> Product/2, Summary1/5  "モータトルク[Nm]"
  [Accel_VDBS] -> Gain/1  "アクセル(%)"
  Subtract1/1 -> Summary1/2  "車両速度　-　目標車速"
  Product/1 -> Summary1/4  "モーターパワー[W]"
  [fuelEfficienty_MPGe] -> トータル電費km/kWh1/1, Summary1/6  "電費　km/kWh"
  [vel_target_kph] -> Mux16/2, Subtract1/2
  Mux16/1 -> Summary1/1  "車両速度（青）/目標車速（紫）"
  m/s to kph/1 -> [vel_target_kph]
  m/s to kph1/1 -> [vel_kph]
  From1/1 -> Gain2/1
  Gain2/1 -> 電費計算1/1(v_vehicle)
  From29/1 -> 電費計算1/2(P_Hi_batt)
  [motor_speed_radPerSec] -> Product/1  "モーター回転数"
  Gain/1 -> Summary1/3  "アクセル(%)"
  Performance Calculations instant/2(L/100Km) -> Terminator1/1
  Performance Calculations instant/1(US MPG) -> Terminator2/1
  Mux1/1 -> [fuelEfficienty_MPGe]
  Abs/1 -> Gain4/1
  Gain4/1 -> Divide/1  "speed_km/h"
  Gain3/1 -> Divide/2  "kWh"
  Divide/1 -> Rate Transition7/1  "km/kWh"
  Rate Transition7/1 -> Mux1/2
  Gain6/1 -> Mux1/1, Performance and FE Scope/6  "電費　km/kWh"

== system TrajectoryFollowVehicleWith14DoF/Variant Subsystem/StanleyControl_vehicleDynamics/Override Z and Pitch/notOverride ==
  currPose : Inport
  Out1 : Outport
  wires:
  currPose/1 -> Out1/1

== system TrajectoryFollowVehicleWith14DoF/Variant Subsystem/StanleyControl_vehicleDynamics/Override Z and Pitch/override ==
  currPose : Inport
  refPose : Inport  Port=2
  Constant : Constant  Value=0
  Mux : Mux  Inputs=3
  Selector : Selector  InputPortWidth=5  IndexOptions=Index vector (dialog)  Indices=[4:5]  OutputSizes=1
  Selector1 : Selector  InputPortWidth=6  IndexOptions=Index vector (dialog)  Indices=1:3  OutputSizes=1
  Selector2 : Selector  NumberOfDimensions=2  InputPortWidth=30  IndexOptions=Index vector (dialog),Select all  Indices=1,1  OutputSizes=1,1
  Out1 : Outport
  wires:
  Mux/1 -> Out1/1
  refPose/1 -> Selector2/1
  currPose/1 -> Selector1/1
  Selector1/1 -> Mux/1
  Selector/1 -> Mux/2
  Constant/1 -> Mux/3
  Selector2/1 -> Selector/1

== system TrajectoryFollowVehicleWith14DoF/Variant Subsystem/StanleyControl_vehicleDynamics/Variant Subsystem/MPC ==
  In Bus Element : Inport  PortName=VehicleInfo  Element=CurrPose
  In Bus Element1 : Inport  PortName=VehicleInfo  Element=CurrVelocity
  RefPose : Inport  Port=2
  Curvature : Inport  Port=3
  Speed : Inport  Port=4
  Constant : Constant  Value=0
  Constant4 : Constant  Value=lr
  Display2 : Display
  Gain1 : Gain  Gain=-1
  Ground : Ground
  MATLAB Function : MATLAB Function  TreatAsAtomicUnit=on
  MATLAB Function1 : MATLAB Function  TreatAsAtomicUnit=on
  MATLAB Function2 : MATLAB Function  TreatAsAtomicUnit=on
  Path Following Control System : mpcadaslib/Path Following Control System  Commented=on  VariantControl=Variant2  ModelType=Use vehicle parameters  VehicleMass=m  VehicleYawInertia=Iz  LengthToFront=lf  LengthToRear=lr  FrontTireStiffness=Cf  RearTireStiffness=Cr  AccelTimeConstant=tau  EgoModelMatrixA=[-2,zeros(1,3);1,zeros(1,3);zeros(1,2),-4.4021,-12.4603;zeros(1,2),1.3913,-5.1868]  EgoModelMatrixB=[2,zeros(1,3);zeros(1,2),24.1270,15.8609]'  EgoModelMatrixC=[zeros(3,1),eye(3)]  InitialLongVel=norm(egoInitialPose.Velocity)  TransportLag=tau2  spaceCtrl=off  DefaultSpacing=0  MinSteering=min_steer  umin_ext=off  MaxSteering=max_steer  umax_ext=off  MinAcceleration=-max_dc  amin_ext=off  MaxAcceleration=max_ac  amax_ext=off  Ts=control_timeStep  PredictionHorizon=PredictionHorizon  ControlHorizon=3  LongWeight=0.1  LateralWeight=1  AccelRateWeight=0.1  SteerRateWeight=0.1  suboptimal=off  maxiter=10  datatypeopt=double  optmode=off  trackmode=off
      settings: LibrarySourceBlock=mpclib/Automated Driving/Path Following Control System
  Path Following wrapper : Subsystem  Variant=on
  Saturation : Saturate  UpperLimit=inf  LowerLimit=0
  Saturation1 : Saturate  UpperLimit=inf  LowerLimit=0
  Saturation2 : Saturate  UpperLimit=inf  LowerLimit=0.01
  Selector : Selector  InputPortWidth=numReferencePose  IndexOptions=Index vector (dialog)  Indices=1  OutputSizes=1
  Selector4 : Selector  InputPortWidth=5  IndexOptions=Index vector (dialog)  Indices=[1:3]  OutputSizes=1
  Selector5 : Selector  InputPortWidth=5  IndexOptions=Index vector (dialog)  Indices=[1:3]  OutputSizes=1
  rad2deg : Gain  Gain=180/pi
  SteerCmd : Outport
  AccelCmd : Outport  Port=2
  DecelCmd : Outport  Port=3
  wires:
  RefPose/1 -> MATLAB Function/1(u)
  In Bus Element/1 -> MATLAB Function1/1(u)
  Constant/1 -> MATLAB Function/2(offset)
  Constant4/1 -> MATLAB Function1/2(offset)
  MATLAB Function/1(y) -> Selector4/1
  MATLAB Function1/1(y) -> Selector5/1
  Path Following wrapper/1(Longitudinal acceleration) -> Gain1/1, Saturation/1
  MATLAB Function2/2(yaw_diff_rad) -> Path Following wrapper/5(Relative yaw angle)
  Selector4/1 -> MATLAB Function2/1(refPose)
  Selector5/1 -> MATLAB Function2/2(currPose)
  Speed/1 -> Selector/1
  In Bus Element1/1 -> Saturation2/1
  MATLAB Function2/1(lateral_deviation) -> Path Following wrapper/4(Lateral deviation)
  Path Following wrapper/2(Steering angle) -> rad2deg/1
  Saturation/1 -> AccelCmd/1
  Saturation1/1 -> DecelCmd/1
  rad2deg/1 -> SteerCmd/1, Display2/1
  Saturation2/1 -> Path Following wrapper/2(Longitudinal velocity)
  Gain1/1 -> Saturation1/1
  Curvature/1 -> Path Following wrapper/3(Curvature)
  Ground/1 -> Path Following wrapper/8(Relative velocity), Path Following wrapper/6(Time gap), Path Following wrapper/7(Relative distance)
  Selector/1 -> Path Following wrapper/1(Set velocity)

== system TrajectoryFollowVehicleWith14DoF/Variant Subsystem/StanleyControl_vehicleDynamics/Variant Subsystem/Stanley ==
  note: x, y, yaw, z, pitch
  In Bus Element : Inport  PortName=VehicleInfo  Element=CurrPose
  In Bus Element1 : Inport  PortName=VehicleInfo  Element=CurrVelocity
  In Bus Element2 : Inport  PortName=VehicleInfo  Element=CurrYawRate
  In Bus Element3 : Inport  PortName=VehicleInfo  Element=CurrSteer
  RefPose : Inport  Port=2
  Curvature : Inport  Port=3
  Speed : Inport  Port=4
  Constant1 : Constant
  Constant2 : Constant
  Constant3 : Constant  Value=0
  Display{,3..5} (4 alike) : Display
  DisplayCurrPose : Display
  DisplayCurrPose1 : Display
  DisplayRefPose : Display
  Lateral Controller Stanley : drivingvehiclecontroller/Lateral Controller Stanley  ModelType=Dynamic bicycle model  PositionGainF=3  PositionGainR=2.5  YawRateGain=0.2  DelayGain=0.2  VehicleMass=m  Lf=lf  Lr=lr  TireStiffness=Cf  Wheelbase=2.8  MaxSteeringAngle=steerLimit
  Longitudinal Controller Stanley : drivingvehiclecontroller/Longitudinal Controller Stanley  Kp=2/2  Ki=1/2  SampleTime=timeStep  MaxAcceleration=max_ac  MaxDeceleration=max_dc
  Saturation : Saturate  UpperLimit=inf  LowerLimit=0.01
  Selector : Selector  InputPortWidth=5  IndexOptions=Index vector (dialog)  Indices=[1:3]  OutputSizes=1
  Selector1 : Selector  InputPortWidth=5  IndexOptions=Index vector (dialog)  Indices=[1:3]  OutputSizes=1
  SteerCmd : Outport
  AccelCmd : Outport  Port=2
  DecelCmd : Outport  Port=3
  wires:
  In Bus Element/1 -> DisplayCurrPose/1, Selector1/1
  In Bus Element3/1 -> Lateral Controller Stanley/7, Display5/1
  In Bus Element2/1 -> Lateral Controller Stanley/6, Display4/1
  In Bus Element1/1 -> Saturation/1
  Constant2/1 -> Lateral Controller Stanley/4
  Selector/1 -> Lateral Controller Stanley/1
  Constant1/1 -> Longitudinal Controller Stanley/3
  Speed/1 -> Longitudinal Controller Stanley/1
  Selector1/1 -> Lateral Controller Stanley/2
  Curvature/1 -> Display3/1, Lateral Controller Stanley/5
  Lateral Controller Stanley/1 -> Display/1, SteerCmd/1
  Longitudinal Controller Stanley/2 -> DecelCmd/1
  Longitudinal Controller Stanley/1 -> AccelCmd/1
  RefPose/1 -> DisplayRefPose/1, Selector/1
  Constant3/1 -> Longitudinal Controller Stanley/4
  Saturation/1 -> DisplayCurrPose1/1, Lateral Controller Stanley/3, Longitudinal Controller Stanley/2

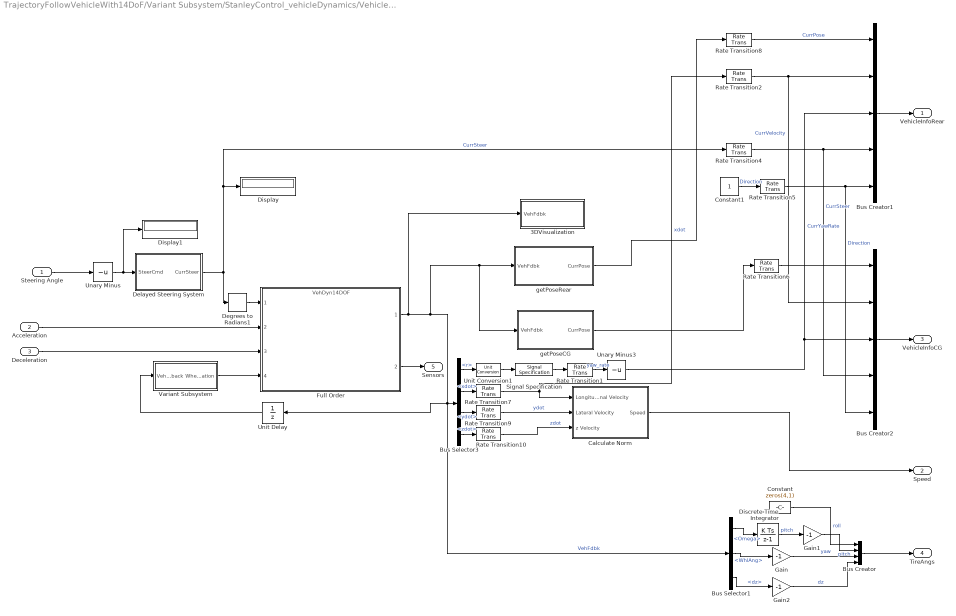
== system TrajectoryFollowVehicleWith14DoF/Variant Subsystem/StanleyControl_vehicleDynamics/Vehicle Dynamics1/Vehicle Dynamics 14DOF ==
  Steering Angle : Inport
  Acceleration : Inport  Port=2
  Deceleration : Inport  Port=3
  3DVisualization : Subsystem  Variant=on
  Bus Creator : BusCreator  Inputs=4
  Bus Creator1 : BusCreator  Inputs=5  OutDataTypeStr=Bus: BusVehicleInfo  NonVirtualBus=on
      settings: InheritFromInputs=off
  Bus Creator2 : BusCreator  Inputs=5  OutDataTypeStr=Bus: BusFullVehicleInfo  NonVirtualBus=on
      settings: InheritFromInputs=off
  Bus Selector1 : BusSelector  OutputSignals=Wheels.TireFrame.Omega,Wheels.Steering.WhlAng,Wheels.TireFrame.dz
  Bus Selector3 : BusSelector  OutputSignals=Body.BdyFrm.Cg.AngVel.r,Body.BdyFrm.Cg.Vel.xdot,Body.BdyFrm.Cg.Vel.ydot,Body.BdyFrm.Cg.Vel.zdot
  Calculate Norm : Subsystem
  Constant : Constant  Value=zeros(4,1)
  Constant1 : Constant
  Degrees to Radians1 : simulink_extras/Transformations/Degrees to Radians
  Delayed Steering System : Subsystem
  Discrete-Time Integrator : DiscreteIntegrator  SampleTime=-1  ICPrevOutput=DiscIntNeverNeededParam  ICPrevScaledInput=DiscIntNeverNeededParam
  Display : Display
  Display1 : Display
  Full Order : ModelReference  ModelNameDialog=VehDyn14DOF.slx  ModelReferenceVersion=8.48
  Gain : Gain  Gain=-1
  Gain1 : Gain  Gain=-1
  Gain2 : Gain  Gain=-1
  Rate Transition{1..2,4..10} (9 alike) : RateTransition  OutPortSampleTime=timeStep
  Signal Specification : SignalSpecification  Unit=deg/s
  Unary Minus : UnaryMinus
  Unary Minus3 : UnaryMinus
  Unit Conversion1 : UnitConversion
  Unit Delay : UnitDelay  SampleTime=-1  HasFrameUpgradeWarning=on
  Variant Subsystem : Subsystem  Variant=on
  getPoseCG : Subsystem
  getPoseRear : Subsystem
  VehicleInfoRear : Outport  VectorParamsAs1DForOutWhenUnconnected=off
  Speed : Outport  Port=2
  VehicleInfoCG : Outport  Port=3  VectorParamsAs1DForOutWhenUnconnected=off
  TireAngs : Outport  Port=4  VectorParamsAs1DForOutWhenUnconnected=off
  Sensors : Outport  Port=5  VectorParamsAs1DForOutWhenUnconnected=off
  wires:
  Calculate Norm/1(Speed) -> Speed/1
  Acceleration/1 -> Full Order/2
  Deceleration/1 -> Full Order/3
  Unary Minus/1 -> Display1/1, Delayed Steering System/1(SteerCmd)
  Degrees to Radians1/1 -> Full Order/1
  Full Order/1 -> 3DVisualization/1(VehFdbk), Bus Selector1/1, Unit Delay/1, Bus Selector3/1, getPoseCG/1(VehFdbk), getPoseRear/1(VehFdbk)  "VehFdbk"
  Variant Subsystem/1(WheelElevation) -> Full Order/4
  Rate Transition9/1 -> Calculate Norm/2(Lateral Velocity)  "ydot"
  Steering Angle/1 -> Unary Minus/1
  Rate Transition1/1 -> Unary Minus3/1  "yaw_rate"
  Delayed Steering System/1(CurrSteer) -> Display/1, Rate Transition4/1, Degrees to Radians1/1  "CurrSteer"
  Unary Minus3/1 -> Bus Creator1/3, Bus Creator2/3  "CurrYawRate"
  Rate Transition5/1 -> Bus Creator2/5, Bus Creator1/5  "Direction"
  Constant1/1 -> Rate Transition5/1  "Direction"
  Rate Transition6/1 -> Bus Creator2/1
  Rate Transition8/1 -> Bus Creator1/1  "CurrPose"
  Bus Creator2/1 -> VehicleInfoCG/1
  Bus Creator1/1 -> VehicleInfoRear/1
  Rate Transition2/1 -> Bus Creator2/2, Bus Creator1/2  "CurrVelocity"
  Rate Transition7/1 -> Calculate Norm/1(Longitudinal Velocity), Rate Transition2/1  "xdot"
  Rate Transition4/1 -> Bus Creator2/4, Bus Creator1/4  "CurrSteer"
  Full Order/2 -> Sensors/1
  Unit Delay/1 -> Variant Subsystem/1(VehFdback)
  Rate Transition10/1 -> Calculate Norm/3(z Velocity)  "zdot"
  Bus Selector3/4 -> Rate Transition10/1  "<zdot>"
  Bus Selector3/3 -> Rate Transition9/1  "<ydot>"
  Unit Conversion1/1 -> Signal Specification/1
  Bus Selector3/2 -> Rate Transition7/1  "<xdot>"
  Bus Selector3/1 -> Unit Conversion1/1  "<r>"
  Signal Specification/1 -> Rate Transition1/1
  getPoseRear/1(CurrPose) -> Rate Transition8/1
  getPoseCG/1(CurrPose) -> Rate Transition6/1
  Gain/1 -> Bus Creator/3  "yaw"
  Bus Creator/1 -> TireAngs/1
  Gain1/1 -> Bus Creator/2  "pitch"
  Constant/1 -> Bus Creator/1  "roll"
  Bus Selector1/2 -> Gain/1  "<WhlAng>"
  Bus Selector1/1 -> Discrete-Time Integrator/1  "<Omega>"
  Discrete-Time Integrator/1 -> Gain1/1  "pitch"
  Bus Selector1/3 -> Gain2/1  "<dz>"
  Gain2/1 -> Bus Creator/4  "dz"
